simulink model "R7014E_QuadTankSim"  (R2025b)
settings: Solver=ode4  StartTime=0.0  StopTime=2000  FixedStep=0.01  RelTol=1e-3  EnableMultiTasking=on
values from neighbouring files (symbols this model uses):
  A1 = 28    [matlab_workspace.mat]
  a1 = 0.071    [matlab_workspace.mat]
  A2 = 32    [matlab_workspace.mat]
  a2 = 0.057    [matlab_workspace.mat]
  A3 = 28    [matlab_workspace.mat]
  a3 = 0.071    [matlab_workspace.mat]
  A4 = 32    [matlab_workspace.mat]
  a4 = 0.057    [matlab_workspace.mat]
  g = 981    [matlab_workspace.mat]
  G11_den = [62.4182361958 1]    [matlab_workspace.mat]
  G11_num = [0 2.59815908165]    [matlab_workspace.mat]
  G22_den = [90.6440624664 1]    [matlab_workspace.mat]
  G22_num = [0 2.84679008684]    [matlab_workspace.mat]
  gamma1 = 0.7    [matlab_workspace.mat]
  gamma1_M = 0.7    [matlab_workspace.mat]
  gamma2 = 0.6    [matlab_workspace.mat]
  gamma2_M = 0.6    [matlab_workspace.mat]
  h1_init = 12.3    [matlab_workspace.mat]
  h2_init = 12.8    [matlab_workspace.mat]
  h3_init = 1.6    [matlab_workspace.mat]
  h4_init = 1.4    [matlab_workspace.mat]
  k1 = 3.33    [matlab_workspace.mat]
  k1_M = 3.33    [matlab_workspace.mat]
  k2 = 3.35    [matlab_workspace.mat]
  k2_M = 3.35    [matlab_workspace.mat]
  Q = gram(G_Pm,'o')    [Gramians_test.m]    (also in matlab_workspace.mat = [1e-08  0  0; 0  1e-08  0; 0  0  10])
  Q11_den = [23.3834317349 15.5889544899 2.59815908165]    [matlab_workspace.mat]
  Q11_num = [0 62.4182361958 1]    [matlab_workspace.mat]
  Q22_den = [25.6211107815 17.080740521 2.84679008684]    [matlab_workspace.mat]
  Q22_num = [0 90.6440624664 1]    [matlab_workspace.mat]
  R = 0.1    [matlab_workspace.mat]
  Ts = 0.02    [matlab_workspace.mat]
undefined symbols (not defined in the file or in its folder): sigbuilder_block
Description:
  | Double tank process simulation model
  | V1.0
  | 
  | Author: Wolfgang Birk, LTU
settings Model: MinMaxOverflowLogging=ForceOff  Creator=wolfgang  LastModifiedBy=kaspe
settings SolverCC: AlgebraicLoopSolver=TrustRegion
settings DataIOCC: LimitDataPoints=on  SaveFormat=Array  SignalLoggingSaveFormat=ModelDataLogs  ReturnWorkspaceOutputs=off
settings OptimizationCC: ExpressionDepthLimit=2147483647.0  LifeSpan=inf
settings DebuggingCC: UnderspecifiedInitializationDetection=Classic  MergeDetectMultiDrivingBlocksExec=none  SolverPrmCheckMsg=warning  FcnCallInpInsideContextMsg=warning  UnconnectedInputMsg=warning  UnconnectedOutputMsg=warning  UnconnectedLineMsg=warning  StateNameClashWarn=warning  SFUnexpectedBacktrackingDiag=warning  SFNoUnconditionalDefaultTransitionDiag=warning  SFExecutionAtInitializationDiag=none  ArithmeticOperatorsInVariantConditions=warning
settings HardwareCC: ProdBitPerPointer=32.0  ProdBitPerSizeT=32.0  ProdBitPerPtrDiffT=32.0  ProdLargestAtomicFloat=None  ProdIntDivRoundTo=Undefined  ProdEndianess=Unspecified  ProdWordSize=32.0  ProdHWDeviceType=32-bit Generic
settings ModelReferenceCC: EnableRefExpFcnMdlSchedulingChecks=on  PropagateSignalLabelsOutOfModel=off
settings SFSimCC: SimUseLocalCustomCode=off  CustomCodeUndefinedFunction=UseInterfaceOnly
settings RTWCC: RTWUseLocalCustomCode=off  GPUComputeCapability=3.5
settings CodeAppCC: StateflowObjectComments=on
settings GRTTargetCC: TargetLangStandard=C89/C90 (ANSI)
settings ConfigComp: CovMetricSettings=dw  CovSaveCumulativeToWorkspaceVar=on  CovSaveSingleToWorkspaceVar=on  CovExternalEMLEnable=off

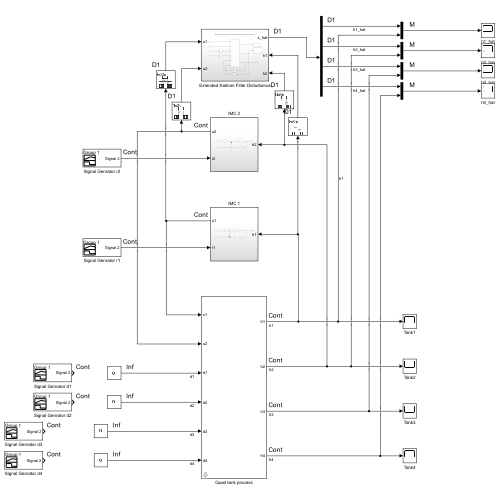
[thumbnail: Simulink's stored preview of the top-level diagram]
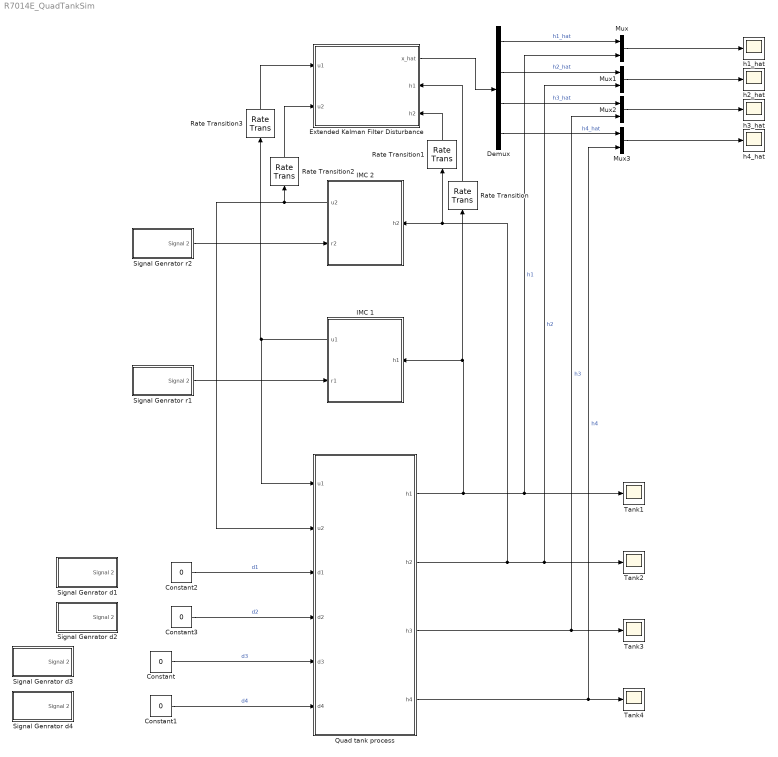
== system R7014E_QuadTankSim ==
  Constant{,1..3} (4 alike) : Constant  Value=0
  Demux : Demux
  Extended Kalman Filter Disturbance : Subsystem
      settings: PortSchema="{\"entries\":[{\"content\":{\"sides\":[{\"content\":{\"connectorIds\":[\"In1\",\"In2\"]},\"type\":\"ConnectorPlacement.EquallySpacedRectSide\",\"uuid\":\"65fe89cb-b391-4b62-a3a2-a3476ef8bc40\"},{\"content\":{\"connectorIds\":[\"Out1\",\"In3\",\"In4\"],\"side\":\"RIGHT\"},\"type\":\"ConnectorPlacement.EquallySpacedRectSide\",\"uuid\":\"bbc6305a-5625-4988-a68f-cd512a800022\"},{\"content\":{\"side\":\"TOP\"},\"type\":\"ConnectorPlacement.EquallySpacedRectSide\",\"uuid\":\"302c5684-92d4-4b6e-95b2-967c1f4e7e8f\"},{\"content\":{\"side\":\"BOTTOM\"},\"type\":\"ConnectorPlacement.EquallySpacedRectSide\",\"uuid\":\"8db0117f-7782-4a07-8d3a-766a48ad4692\"}]},\"type\":\"ConnectorPlacement.EquallySpacedConnector\",\"uuid\":\"a95b63f5-df7a-433e-a941-cc1845937f8d\"}],\"packageUris\":[\"http://schema.mathworks.com/mf0/Connector/R2020b\"],\"version\":\"1.0\"}"
  IMC 1 : Subsystem
      settings: PortSchema="{\"entries\":[{\"content\":{\"sides\":[{\"content\":{\"connectorIds\":[\"In1\"]},\"type\":\"ConnectorPlacement.EquallySpacedRectSide\",\"uuid\":\"4852cb48-3dbe-49d3-b52d-1f2b66e5782f\"},{\"content\":{\"connectorIds\":[\"Out1\",\"In2\"],\"side\":\"RIGHT\"},\"type\":\"ConnectorPlacement.EquallySpacedRectSide\",\"uuid\":\"9cc98c43-55ba-47ec-98d3-91ba0e651a74\"},{\"content\":{\"side\":\"TOP\"},\"type\":\"ConnectorPlacement.EquallySpacedRectSide\",\"uuid\":\"0e4ead2b-996b-4075-849e-a6886983cab4\"},{\"content\":{\"side\":\"BOTTOM\"},\"type\":\"ConnectorPlacement.EquallySpacedRectSide\",\"uuid\":\"443cd1da-2b11-4b7b-ba12-e267a6b444a4\"}]},\"type\":\"ConnectorPlacement.EquallySpacedConnector\",\"uuid\":\"d0829c27-0885-4d8f-a753-a80de6d2ea12\"}],\"packageUris\":[\"http://schema.mathworks.com/mf0/Connector/R2020b\"],\"version\":\"1.0\"}"
  IMC 2 : Subsystem
      settings: PortSchema="{\"entries\":[{\"content\":{\"sides\":[{\"content\":{\"connectorIds\":[\"In1\"]},\"type\":\"ConnectorPlacement.EquallySpacedRectSide\",\"uuid\":\"4852cb48-3dbe-49d3-b52d-1f2b66e5782f\"},{\"content\":{\"connectorIds\":[\"Out1\",\"In2\"],\"side\":\"RIGHT\"},\"type\":\"ConnectorPlacement.EquallySpacedRectSide\",\"uuid\":\"9cc98c43-55ba-47ec-98d3-91ba0e651a74\"},{\"content\":{\"side\":\"TOP\"},\"type\":\"ConnectorPlacement.EquallySpacedRectSide\",\"uuid\":\"0e4ead2b-996b-4075-849e-a6886983cab4\"},{\"content\":{\"side\":\"BOTTOM\"},\"type\":\"ConnectorPlacement.EquallySpacedRectSide\",\"uuid\":\"84a55638-02cd-431e-8938-8d2f80adb47b\"}]},\"type\":\"ConnectorPlacement.EquallySpacedConnector\",\"uuid\":\"d0829c27-0885-4d8f-a753-a80de6d2ea12\"}],\"packageUris\":[\"http://schema.mathworks.com/mf0/Connector/R2020b\"],\"version\":\"1.0\"}"
  Mux{,1..3} (4 alike) : Mux  Inputs=2
  Quad tank process : Subsystem  mask{hmax=20, A1=A1, ao1=a1, h10=0, A2=A2, ao2=a2, h20=0, A3=A3, ao3=a3, h30=0, A4=A4, ao4=a4, h40=0, k1=k1_M, k2=k2_M, gamma1=gamma1_M, gamma2=gamma2_M}
      mask prompts: hmax "Tank height (cm)"; A1 "Tank area (cm^2)"; ao1 "Opening area (cm^2)"; h10 "Initial level (cm)"; A2 "Tank area (cm^2)"; ao2 "Opening area (cm^2)"; h20 "Initial level (cm)"; A3 "Tank area (cm^2)"; ao3 "Opening area (cm^2)"; h30 "Initial level (cm)"; A4 "Tank area (cm^2)"; ao4 "Opening area (cm^2)"; h40 "Initial level (cm)"; k1 "Pump1 gain (cm^3/V/s)"; k2 "Pump2 gain (cm^3/V/s)"; gamma1 "Split valve gamma 1"; gamma2 "Split valve gamma 2"
      mask help: Double tank process parameters
      mask DialogControl Container3 Prompt: General parameters
      mask DialogControl ParameterGroupVar Prompt: Tank 1
      mask DialogControl ParameterGroupVar_copy_copy_copy Prompt: Tank 2
      mask DialogControl ParameterGroupVar_copy_copy Prompt: Tank 3
      mask DialogControl ParameterGroupVar_copy Prompt: Tank 4
      mask DialogControl Container4 Prompt: Pump parameters
  Rate Transition : RateTransition  InitialCondition=h1_init  OutPortSampleTime=Ts
  Rate Transition1 : RateTransition  InitialCondition=h2_init  OutPortSampleTime=Ts
  Rate Transition2 : RateTransition  InitialCondition=h2_init  OutPortSampleTime=Ts
  Rate Transition3 : RateTransition  InitialCondition=h2_init  OutPortSampleTime=Ts
  Signal Genrator d1 : Subsystem  Tag=STV Subsys  LoadFcn=sigbuilder_block('load');  StartFcn=sigbuilder_block('start');  StopFcn=sigbuilder_block('stop');  ClipboardFcn=sigbuilder_block('clipboard');  mask(Sigbuilder block){tuvar=[0:10]}
      mask help: Simulink:masks:SigbuilderBlock_MD
      mask init:
      | if ~strcmp(get_param(bdroot(gcbh),'SimulationStatus'),'stopped') tuvar = sigbuilder_block('maskInit'); end
      settings: CopyFcn=sigbuilder_block('copy');  DeleteFcn=sigbuilder_block('delete');  ModelCloseFcn=sigbuilder_block('modelClose');  PreSaveFcn=sigbuilder_block('preSave');  PauseFcn=sigbuilder_block('pause');  ContinueFcn=sigbuilder_block('continue');  NameChangeFcn=sigbuilder_block('namechange');  OpenFcn=sigbuilder_block('open',[335.25 1257.75 630.75 369 ]);  CloseFcn=sigbuilder_block('close');
      mask Display: plot(0, 0, 100, 100,[2, 2, 32, 32, 2], [68, 8, 8, 68, 68],[32, 2], [38, 38], [32, 19, 2],[53, 60, 44], [32, 17, 17, 2],[16, 16, 31, 31]);txt = getActiveGroup(gcbh);text(2, 100, txt,'verticalAlignment', 'top');
  Signal Genrator d2 : Subsystem  Tag=STV Subsys  LoadFcn=sigbuilder_block('load');  StartFcn=sigbuilder_block('start');  StopFcn=sigbuilder_block('stop');  ClipboardFcn=sigbuilder_block('clipboard');  mask(Sigbuilder block){tuvar=[0:10]}
      mask help: Simulink:masks:SigbuilderBlock_MD
      mask init:
      | if ~strcmp(get_param(bdroot(gcbh),'SimulationStatus'),'stopped') tuvar = sigbuilder_block('maskInit'); end
      settings: CopyFcn=sigbuilder_block('copy');  DeleteFcn=sigbuilder_block('delete');  ModelCloseFcn=sigbuilder_block('modelClose');  PreSaveFcn=sigbuilder_block('preSave');  PauseFcn=sigbuilder_block('pause');  ContinueFcn=sigbuilder_block('continue');  NameChangeFcn=sigbuilder_block('namechange');  OpenFcn=sigbuilder_block('open',[609.75 1396.5 630.75 369 ]);  CloseFcn=sigbuilder_block('close');
      mask Display: plot(0, 0, 100, 100,[2, 2, 32, 32, 2], [68, 8, 8, 68, 68],[32, 2], [38, 38], [32, 19, 2],[53, 60, 44], [32, 17, 17, 2],[16, 16, 31, 31]);txt = getActiveGroup(gcbh);text(2, 100, txt,'verticalAlignment', 'top');
  Signal Genrator d3 : Subsystem  Tag=STV Subsys  LoadFcn=sigbuilder_block('load');  StartFcn=sigbuilder_block('start');  StopFcn=sigbuilder_block('stop');  ClipboardFcn=sigbuilder_block('clipboard');  mask(Sigbuilder block){tuvar=[0:10]}
      mask help: Simulink:masks:SigbuilderBlock_MD
      mask init:
      | if ~strcmp(get_param(bdroot(gcbh),'SimulationStatus'),'stopped') tuvar = sigbuilder_block('maskInit'); end
      settings: CopyFcn=sigbuilder_block('copy');  DeleteFcn=sigbuilder_block('delete');  ModelCloseFcn=sigbuilder_block('modelClose');  PreSaveFcn=sigbuilder_block('preSave');  PauseFcn=sigbuilder_block('pause');  ContinueFcn=sigbuilder_block('continue');  NameChangeFcn=sigbuilder_block('namechange');  OpenFcn=sigbuilder_block('open',[603.75 1322.25 630.75 369 ]);  CloseFcn=sigbuilder_block('close');
      mask Display: plot(0, 0, 100, 100,[2, 2, 32, 32, 2], [68, 8, 8, 68, 68],[32, 2], [38, 38], [32, 19, 2],[53, 60, 44], [32, 17, 17, 2],[16, 16, 31, 31]);txt = getActiveGroup(gcbh);text(2, 100, txt,'verticalAlignment', 'top');
  Signal Genrator d4 : Subsystem  Tag=STV Subsys  LoadFcn=sigbuilder_block('load');  StartFcn=sigbuilder_block('start');  StopFcn=sigbuilder_block('stop');  ClipboardFcn=sigbuilder_block('clipboard');  mask(Sigbuilder block){tuvar=[0:10]}
      mask help: Simulink:masks:SigbuilderBlock_MD
      mask init:
      | if ~strcmp(get_param(bdroot(gcbh),'SimulationStatus'),'stopped') tuvar = sigbuilder_block('maskInit'); end
      settings: CopyFcn=sigbuilder_block('copy');  DeleteFcn=sigbuilder_block('delete');  ModelCloseFcn=sigbuilder_block('modelClose');  PreSaveFcn=sigbuilder_block('preSave');  PauseFcn=sigbuilder_block('pause');  ContinueFcn=sigbuilder_block('continue');  NameChangeFcn=sigbuilder_block('namechange');  OpenFcn=sigbuilder_block('open',[271.5 378 630.75 369 ]);  CloseFcn=sigbuilder_block('close');
      mask Display: plot(0, 0, 100, 100,[2, 2, 32, 32, 2], [68, 8, 8, 68, 68],[32, 2], [38, 38], [32, 19, 2],[53, 60, 44], [32, 17, 17, 2],[16, 16, 31, 31]);txt = getActiveGroup(gcbh);text(2, 100, txt,'verticalAlignment', 'top');
  Signal Genrator r1 : Subsystem  Tag=STV Subsys  LoadFcn=sigbuilder_block('load');  StartFcn=sigbuilder_block('start');  StopFcn=sigbuilder_block('stop');  ClipboardFcn=sigbuilder_block('clipboard');  mask(Sigbuilder block){tuvar=[0:10]}
      mask help: Simulink:masks:SigbuilderBlock_MD
      mask init:
      | if ~strcmp(get_param(bdroot(gcbh),'SimulationStatus'),'stopped') tuvar = sigbuilder_block('maskInit'); end
      settings: CopyFcn=sigbuilder_block('copy');  DeleteFcn=sigbuilder_block('delete');  ModelCloseFcn=sigbuilder_block('modelClose');  PreSaveFcn=sigbuilder_block('preSave');  PauseFcn=sigbuilder_block('pause');  ContinueFcn=sigbuilder_block('continue');  NameChangeFcn=sigbuilder_block('namechange');  OpenFcn=sigbuilder_block('open',[271.5 378 630.75 369 ]);  CloseFcn=sigbuilder_block('close');
      mask Display: plot(0, 0, 100, 100,[2, 2, 32, 32, 2], [68, 8, 8, 68, 68],[32, 2], [38, 38], [32, 19, 2],[53, 60, 44], [32, 17, 17, 2],[16, 16, 31, 31]);txt = getActiveGroup(gcbh);text(2, 100, txt,'verticalAlignment', 'top');
  Signal Genrator r2 : Subsystem  Tag=STV Subsys  LoadFcn=sigbuilder_block('load');  StartFcn=sigbuilder_block('start');  StopFcn=sigbuilder_block('stop');  ClipboardFcn=sigbuilder_block('clipboard');  mask(Sigbuilder block){tuvar=[0:10]}
      mask help: Simulink:masks:SigbuilderBlock_MD
      mask init:
      | if ~strcmp(get_param(bdroot(gcbh),'SimulationStatus'),'stopped') tuvar = sigbuilder_block('maskInit'); end
      settings: CopyFcn=sigbuilder_block('copy');  DeleteFcn=sigbuilder_block('delete');  ModelCloseFcn=sigbuilder_block('modelClose');  PreSaveFcn=sigbuilder_block('preSave');  PauseFcn=sigbuilder_block('pause');  ContinueFcn=sigbuilder_block('continue');  NameChangeFcn=sigbuilder_block('namechange');  OpenFcn=sigbuilder_block('open',[271.5 378 630.75 369 ]);  CloseFcn=sigbuilder_block('close');
      mask Display: plot(0, 0, 100, 100,[2, 2, 32, 32, 2], [68, 8, 8, 68, 68],[32, 2], [38, 38], [32, 19, 2],[53, 60, 44], [32, 17, 17, 2],[16, 16, 31, 31]);txt = getActiveGroup(gcbh);text(2, 100, txt,'verticalAlignment', 'top');
  Tank{1..4} (4 alike) : Scope
      Tank1 settings: TimeSpan=100  ActiveDisplayYMinimum=-1.8059795256397659  ActiveDisplayYMaximum=16.253815730757896
      Tank2 settings: TimeSpan=100  ActiveDisplayYMinimum=-1.9584679823736892  ActiveDisplayYMaximum=17.626211841363208  DataLoggingVariableName=ScopeData3
      Tank3 settings: TimeSpan=100  ActiveDisplayYMinimum=1.57505  ActiveDisplayYMaximum=1.66866
      Tank4 settings: TimeSpan=100  ActiveDisplayYMinimum=1.35987  ActiveDisplayYMaximum=1.45363  DataLoggingVariableName=ScopeData2
  h1_hat : Scope
      settings: ActiveDisplayYMinimum=-1.8062354240144811  ActiveDisplayYMaximum=16.256118816130336  DataLoggingVariableName=ScopeData4
  h2_hat : Scope
      settings: ActiveDisplayYMinimum=-1.8062354240144811  ActiveDisplayYMaximum=16.256118816130336  DataLoggingVariableName=ScopeData5
  h3_hat : Scope
      settings: ActiveDisplayYMinimum=-1.8062354240144811  ActiveDisplayYMaximum=16.256118816130336  DataLoggingVariableName=ScopeData6
  h4_hat : Scope
      settings: ActiveDisplayYMinimum=-1.8062354240144811  ActiveDisplayYMaximum=16.256118816130336  DataLoggingVariableName=ScopeData7
  wires:
  Quad tank process/3(h3) -> Mux2/2, Tank3/1  "h3"
  Quad tank process/1(h1) -> IMC 1/1(h1), Rate Transition/1, Mux/2, Tank1/1  "h1"
  Constant2/1 -> Quad tank process/3(d1)  "d1"
  Constant3/1 -> Quad tank process/4(d2)  "d2"
  Constant/1 -> Quad tank process/5(d3)  "d3"
  Constant1/1 -> Quad tank process/6(d4)  "d4"
  Quad tank process/2(h2) -> Mux1/2, Tank2/1, IMC 2/1(h2), Rate Transition1/1  "h2"
  Quad tank process/4(h4) -> Mux3/2, Tank4/1  "h4"
  IMC 1/1(u1) -> Rate Transition3/1, Quad tank process/1(u1)
  Signal Genrator r1/1(Signal 2) -> IMC 1/2(r1)
  Signal Genrator r2/1(Signal 2) -> IMC 2/2(r2)
  IMC 2/1(u2) -> Quad tank process/2(u2), Rate Transition2/1
  Rate Transition/1 -> Extended Kalman Filter Disturbance/3(h1)
  Rate Transition1/1 -> Extended Kalman Filter Disturbance/4(h2)
  Rate Transition2/1 -> Extended Kalman Filter Disturbance/2(u2)
  Rate Transition3/1 -> Extended Kalman Filter Disturbance/1(u1)
  Extended Kalman Filter Disturbance/1(x_hat) -> Demux/1
  Demux/1 -> Mux/1  "h1_hat"
  Mux/1 -> h1_hat/1
  Demux/2 -> Mux1/1  "h2_hat"
  Demux/3 -> Mux2/1  "h3_hat"
  Demux/4 -> Mux3/1  "h4_hat"
  Mux1/1 -> h2_hat/1
  Mux2/1 -> h3_hat/1
  Mux3/1 -> h4_hat/1

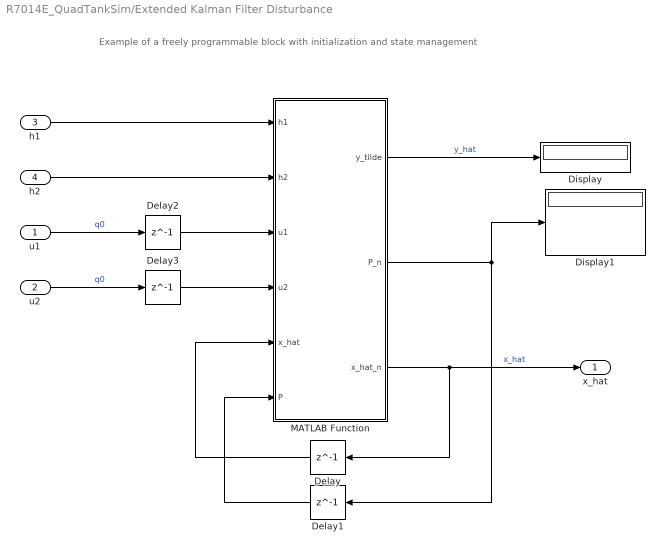
== system R7014E_QuadTankSim/Extended Kalman Filter Disturbance ==
  note: Example of a freely programmable block with initialization and state management
  u1 : Inport
  u2 : Inport  Port=2
  h1 : Inport  Port=3
  h2 : Inport  Port=4
  Delay : Delay  DelayLength=1  InitialCondition=[h1_init, h2_init, h3_init, h4_init]
  Delay1 : Delay  DelayLength=1  InitialCondition=zeros(4)
  Delay2 : Delay  DelayLength=1  InitialCondition=0
  Delay3 : Delay  DelayLength=1  InitialCondition=0
  Display : Display
  Display1 : Display
  MATLAB Function : MATLAB Function  TreatAsAtomicUnit=on
  x_hat : Outport
  wires:
  Delay/1 -> MATLAB Function/5(x_hat)
  MATLAB Function/1(y_tilde) -> Display/1  "y_hat"
  MATLAB Function/2(P_n) -> Display1/1, Delay1/1
  Delay1/1 -> MATLAB Function/6(P)
  u1/1 -> Delay2/1  "q0"
  MATLAB Function/3(x_hat_n) -> x_hat/1, Delay/1  "x_hat"
  Delay2/1 -> MATLAB Function/3(u1)
  Delay3/1 -> MATLAB Function/4(u2)
  u2/1 -> Delay3/1  "q0"
  h2/1 -> MATLAB Function/2(h2)
  h1/1 -> MATLAB Function/1(h1)

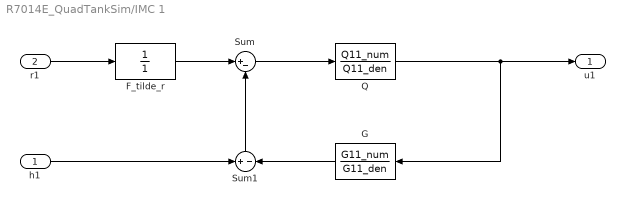
== system R7014E_QuadTankSim/IMC 1 ==
  h1 : Inport
  r1 : Inport  Port=2
  F_tilde_r : TransferFcn  Denominator=[1]
  G : TransferFcn  Numerator=G11_num  Denominator=G11_den
  Q : TransferFcn  Numerator=Q11_num  Denominator=Q11_den
  Sum : Sum  Inputs=|+-
  Sum1 : Sum  Inputs=+|-
  u1 : Outport
  wires:
  F_tilde_r/1 -> Sum/1
  r1/1 -> F_tilde_r/1
  Sum/1 -> Q/1
  Sum1/1 -> Sum/2
  Q/1 -> G/1, u1/1
  G/1 -> Sum1/2
  h1/1 -> Sum1/1

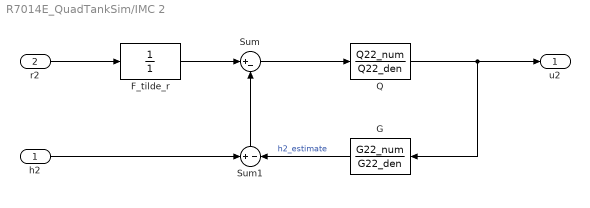
== system R7014E_QuadTankSim/IMC 2 ==
  h2 : Inport
  r2 : Inport  Port=2
  F_tilde_r : TransferFcn  Denominator=[1]
  G : TransferFcn  Numerator=G22_num  Denominator=G22_den
  Q : TransferFcn  Numerator=Q22_num  Denominator=Q22_den
  Sum : Sum  Inputs=|+-
  Sum1 : Sum  Inputs=+|-
  u2 : Outport
  wires:
  F_tilde_r/1 -> Sum/1
  r2/1 -> F_tilde_r/1
  Sum/1 -> Q/1
  Sum1/1 -> Sum/2
  Q/1 -> u2/1, G/1
  h2/1 -> Sum1/1
  G/1 -> Sum1/2  "h2_estimate"

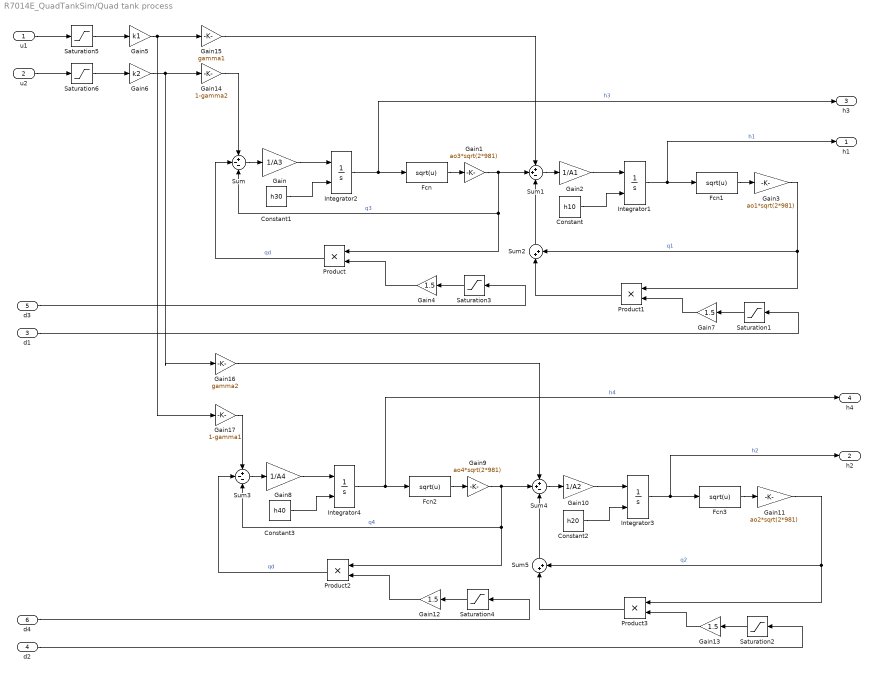
== system R7014E_QuadTankSim/Quad tank process ==
  u1 : Inport
  u2 : Inport  Port=2
  d1 : Inport  Port=3
  d2 : Inport  Port=4
  d3 : Inport  Port=5
  d4 : Inport  Port=6
  Constant : Constant  Value=h10
  Constant1 : Constant  Value=h30
  Constant2 : Constant  Value=h20
  Constant3 : Constant  Value=h40
  Fcn{,1..3} (4 alike) : Fcn  Expr=sqrt(u)
  Gain : Gain  Gain=1/A3
  Gain1 : Gain  Gain=ao3*sqrt(2*981)
  Gain10 : Gain  Gain=1/A2
  Gain11 : Gain  Gain=ao2*sqrt(2*981)
  Gain{4,7,12..13} (4 alike) : Gain  Gain=1.5
  Gain14 : Gain  Gain=1-gamma2
  Gain15 : Gain  Gain=gamma1
  Gain16 : Gain  Gain=gamma2
  Gain17 : Gain  Gain=1-gamma1
  Gain2 : Gain  Gain=1/A1
  Gain3 : Gain  Gain=ao1*sqrt(2*981)
  Gain5 : Gain  Gain=k1
  Gain6 : Gain  Gain=k2
  Gain8 : Gain  Gain=1/A4
  Gain9 : Gain  Gain=ao4*sqrt(2*981)
  Integrator{1..4} (4 alike) : Integrator  InitialConditionSource=external  LimitOutput=on  UpperSaturationLimit=hmax  LowerSaturationLimit=0
  Product{,1..3} (4 alike) : Product  RndMeth=Zero
  Saturation{1..4} (4 alike) : Saturate  UpperLimit=1  LowerLimit=0
  Saturation5 : Saturate  UpperLimit=10  LowerLimit=0
  Saturation6 : Saturate  UpperLimit=10  LowerLimit=0
  Sum : Sum  Inputs=+--
  Sum1 : Sum  Inputs=++-
  Sum2 : Sum  Inputs=|++
  Sum3 : Sum  Inputs=+--
  Sum4 : Sum  Inputs=++-
  Sum5 : Sum  Inputs=|++
  h1 : Outport  VectorParamsAs1DForOutWhenUnconnected=off
  h2 : Outport  Port=2  VectorParamsAs1DForOutWhenUnconnected=off
  h3 : Outport  Port=3  VectorParamsAs1DForOutWhenUnconnected=off
  h4 : Outport  Port=4  VectorParamsAs1DForOutWhenUnconnected=off
  wires:
  Sum/1 -> Gain/1
  Gain/1 -> Integrator2/1
  Fcn/1 -> Gain1/1
  Gain1/1 -> Product/1, Sum/3, Sum1/2  "q3"
  Sum1/1 -> Gain2/1
  Gain2/1 -> Integrator1/1
  Fcn1/1 -> Gain3/1
  Integrator2/1 -> h3/1, Fcn/1  "h3"
  Product/1 -> Sum/2  "qd"
  d3/1 -> Saturation3/1
  Integrator1/1 -> h1/1, Fcn1/1  "h1"
  Saturation3/1 -> Gain4/1
  Gain4/1 -> Product/2
  u1/1 -> Saturation5/1
  Constant/1 -> Integrator1/2
  Constant1/1 -> Integrator2/2
  u2/1 -> Saturation6/1
  Gain5/1 -> Gain17/1, Gain15/1
  Sum2/1 -> Sum1/3
  Gain3/1 -> Product1/1, Sum2/2  "q1"
  Gain7/1 -> Product1/2
  Saturation1/1 -> Gain7/1
  d1/1 -> Saturation1/1
  Product1/1 -> Sum2/1
  Product3/1 -> Sum5/1
  d2/1 -> Saturation2/1
  Saturation2/1 -> Gain13/1
  Gain13/1 -> Product3/2
  Gain11/1 -> Sum5/2, Product3/1  "q2"
  Sum5/1 -> Sum4/3
  Constant3/1 -> Integrator4/2
  Constant2/1 -> Integrator3/2
  Gain12/1 -> Product2/2
  Saturation4/1 -> Gain12/1
  Integrator3/1 -> Fcn3/1, h2/1  "h2"
  d4/1 -> Saturation4/1
  Product2/1 -> Sum3/2  "qd"
  Integrator4/1 -> h4/1, Fcn2/1  "h4"
  Fcn3/1 -> Gain11/1
  Gain10/1 -> Integrator3/1
  Sum4/1 -> Gain10/1
  Gain9/1 -> Sum4/2, Sum3/3, Product2/1  "q4"
  Fcn2/1 -> Gain9/1
  Gain8/1 -> Integrator4/1
  Sum3/1 -> Gain8/1
  Gain14/1 -> Sum/1
  Gain15/1 -> Sum1/1
  Gain6/1 -> Gain16/1, Gain14/1
  Gain16/1 -> Sum4/1
  Gain17/1 -> Sum3/1
  Saturation5/1 -> Gain5/1
  Saturation6/1 -> Gain6/1

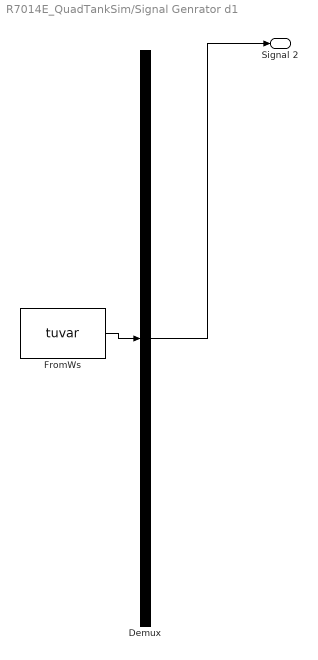
== system R7014E_QuadTankSim/Signal Genrator d1 ==
  Demux : Demux  Tag=STV Demux  Outputs=1
      settings: DisplayOption=none
  FromWs : FromWorkspace  Tag=STV FromWs  VariableName=tuvar
      SigBuilderData=|
      | common.afterFinalStr = 'Extrapolate'
      | common.sampleTime = 0
      | dataSet.timeRange = [0 2000]
      | dataSet.name = 'Group 1'
      | sbobj.Groups.Name = 'Group 1'
      | sbobj.Groups.Signals.Name = 'Signal 2'
      | sbobj.Groups.Signals.XData = [0 1400 1400 2000]
      | sbobj.Groups.Signals.YData = [0.5 0.5 0.75 0.75]
      | sbobj.Groups.TimeRange = [0 2000]
  Signal 2 : Outport  Tag=STV Outport
  wires:
  FromWs/1 -> Demux/1
  Demux/1 -> Signal 2/1

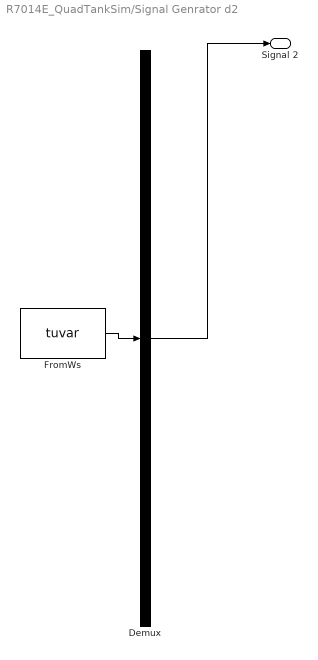
== system R7014E_QuadTankSim/Signal Genrator d2 ==
  Demux : Demux  Tag=STV Demux  Outputs=1
      settings: DisplayOption=none
  FromWs : FromWorkspace  Tag=STV FromWs  VariableName=tuvar
      SigBuilderData=|
      | common.afterFinalStr = 'Extrapolate'
      | common.sampleTime = 0
      | dataSet.timeRange = [0 2000]
      | dataSet.name = 'Group 1'
      | sbobj.Groups.Name = 'Group 1'
      | sbobj.Groups.Signals.Name = 'Signal 2'
      | sbobj.Groups.Signals.XData = [0 1400 1400 2000]
      | sbobj.Groups.Signals.YData = [0.5 0.5 0.25 0.25]
      | sbobj.Groups.TimeRange = [0 2000]
  Signal 2 : Outport  Tag=STV Outport
  wires:
  FromWs/1 -> Demux/1
  Demux/1 -> Signal 2/1

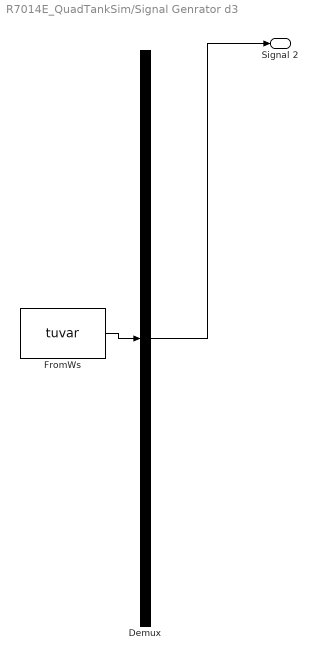
== system R7014E_QuadTankSim/Signal Genrator d3 ==
  Demux : Demux  Tag=STV Demux  Outputs=1
      settings: DisplayOption=none
  FromWs : FromWorkspace  Tag=STV FromWs  VariableName=tuvar
      SigBuilderData=|
      | common.afterFinalStr = 'Extrapolate'
      | common.sampleTime = 0
      | dataSet.timeRange = [0 2000]
      | dataSet.name = 'Group 1'
      | sbobj.Groups.Name = 'Group 1'
      | sbobj.Groups.Signals.Name = 'Signal 2'
      | sbobj.Groups.Signals.XData = [0 800 800 2000]
      | sbobj.Groups.Signals.YData = [12.3 12.3 14.3 14.3]
      | sbobj.Groups.TimeRange = [0 2000]
  Signal 2 : Outport  Tag=STV Outport
  wires:
  FromWs/1 -> Demux/1
  Demux/1 -> Signal 2/1

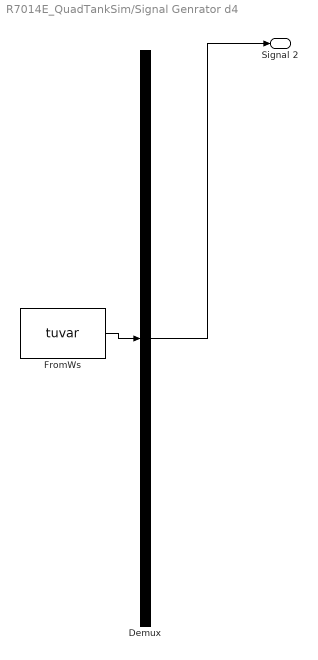
== system R7014E_QuadTankSim/Signal Genrator d4 ==
  Demux : Demux  Tag=STV Demux  Outputs=1
      settings: DisplayOption=none
  FromWs : FromWorkspace  Tag=STV FromWs  VariableName=tuvar
      SigBuilderData=|
      | common.afterFinalStr = 'Extrapolate'
      | common.sampleTime = 0
      | dataSet.timeRange = [0 2000]
      | dataSet.name = 'Group 1'
      | sbobj.Groups.Name = 'Group 1'
      | sbobj.Groups.Signals.Name = 'Signal 2'
      | sbobj.Groups.Signals.XData = [0 800 800 2000]
      | sbobj.Groups.Signals.YData = [12.3 12.3 14.3 14.3]
      | sbobj.Groups.TimeRange = [0 2000]
  Signal 2 : Outport  Tag=STV Outport
  wires:
  FromWs/1 -> Demux/1
  Demux/1 -> Signal 2/1

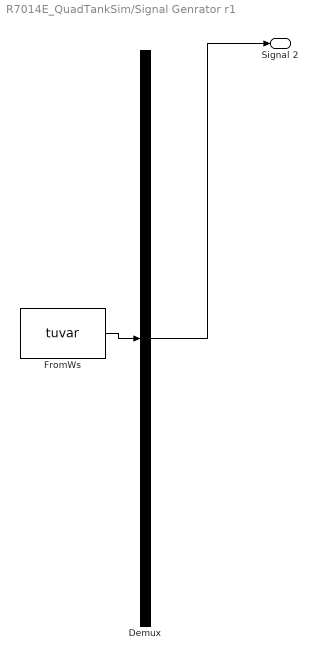
== system R7014E_QuadTankSim/Signal Genrator r1 ==
  Demux : Demux  Tag=STV Demux  Outputs=1
      settings: DisplayOption=none
  FromWs : FromWorkspace  Tag=STV FromWs  VariableName=tuvar
      SigBuilderData=|
      | common.afterFinalStr = 'Extrapolate'
      | common.sampleTime = 0
      | dataSet.timeRange = [0 2000]
      | dataSet.name = 'Group 1'
      | sbobj.Groups.Name = 'Group 1'
      | sbobj.Groups.Signals.Name = 'Signal 2'
      | sbobj.Groups.Signals.XData = [0 800 800 2000]
      | sbobj.Groups.Signals.YData = [12.3 12.3 14.3 14.3]
      | sbobj.Groups.TimeRange = [0 2000]
  Signal 2 : Outport  Tag=STV Outport
  wires:
  FromWs/1 -> Demux/1
  Demux/1 -> Signal 2/1

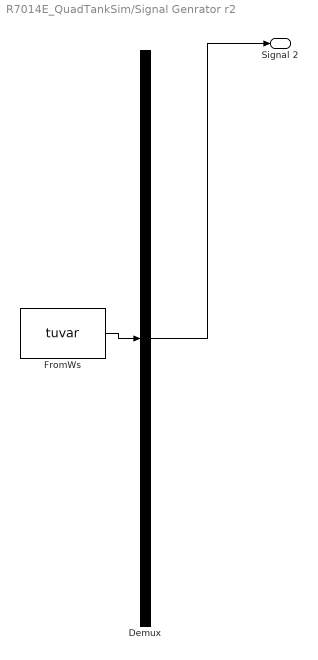
== system R7014E_QuadTankSim/Signal Genrator r2 ==
  Demux : Demux  Tag=STV Demux  Outputs=1
      settings: DisplayOption=none
  FromWs : FromWorkspace  Tag=STV FromWs  VariableName=tuvar
      SigBuilderData=|
      | common.afterFinalStr = 'Extrapolate'
      | common.sampleTime = 0
      | dataSet.timeRange = [0 2000]
      | dataSet.name = 'Group 1'
      | sbobj.Groups.Name = 'Group 1'
      | sbobj.Groups.Signals.Name = 'Signal 2'
      | sbobj.Groups.Signals.XData = [0 800 800 2000]
      | sbobj.Groups.Signals.YData = [12.8 12.8 14.8 14.8]
      | sbobj.Groups.TimeRange = [0 2000]
  Signal 2 : Outport  Tag=STV Outport
  wires:
  FromWs/1 -> Demux/1
  Demux/1 -> Signal 2/1

== matlab function R7014E_QuadTankSim/Extended Kalman Filter Disturbance/MATLAB Function ==
  data: h1 input; h2 input; u1 input; u2 input; x_hat input; y_tilde output; P input; P_n output; x_hat_n output; Q parameter; R parameter; g parameter; Ts parameter; A1 parameter; A2 parameter; A3 parameter; A4 parameter; k1 parameter; k2 parameter; a1 parameter; a2 parameter; a3 parameter; a4 parameter; gamma1 parameter; gamma2 parameter
function [y_tilde, P_n, x_hat_n] = fcn(h1, h2, u1, u2, x_hat, P, Q, R, g, Ts, A1, A2, A3, A4, k1, k2, a1, a2, a3, a4, gamma1, gamma2)

h1_hat = x_hat(1);
h2_hat = x_hat(2);
h3_hat = x_hat(3);
h4_hat = x_hat(4);
Q = eye(4);
% Linearization


% Disturbances (Assumed zero for the filter's internal model unless estimated)
d1 = 0; d2 = 0; d3 = 0; d4 = 0;

% Safety margin to prevent division by zero if a tank empties
epsilon = 1e-6; 

%% Calculate State Jacobian Matrix (A)
A = zeros(4, 4);

A(1,1) = -((a1 + d1) / A1) * sqrt(g / (2 * max(h1_hat, epsilon)));
A(1,3) =  (a3 / A3) * sqrt(g / (2 * max(h3_hat, epsilon)));

A(2,2) = -((a2 + d2) / A2) * sqrt(g / (2 * max(h2_hat, epsilon)));
A(2,4) =  (a4 / A4) * sqrt(g / (2 * max(h4_hat, epsilon)));

A(3,3) = -((a3 + d3) / A3) * sqrt(g / (2 * max(h3_hat, epsilon)));

A(4,4) = -((a4 + d4) / A4) * sqrt(g / (2 * max(h4_hat, epsilon)));

%% Calculate Input Jacobian Matrix (B)
B = zeros(4, 2);

B(1,1) = (gamma1 * k1) / A1;
B(2,2) = (gamma2 * k2) / A2;
B(3,2) = ((1 - gamma2) * k2) / A3;
B(4,1) = ((1 - gamma1) * k1) / A4;

Ad = eye(size(A)) + Ts * A;

% Predict
sqrt1 = sqrt(2*g*max(h1_hat, epsilon));
sqrt2 = sqrt(2*g*max(h2_hat, epsilon));
sqrt3 = sqrt(2*g*max(h3_hat, epsilon));
sqrt4 = sqrt(2*g*max(h4_hat, epsilon));
x_hat_dot = [(-a1-d1)/A1*sqrt1+a3/A3*sqrt3+gamma1/A1*k1*u1;
             (-a2-d2)/A2*sqrt2+a4/A4*sqrt4+gamma2/A2*k2*u2;
             (-a3-d3)/A3*sqrt3+(1-gamma2)/A3*k2*u2;
             (-a4-d4)/A4*sqrt4+(1-gamma1)/A4*k1*u1;];
x_hat_n = x_hat + x_hat_dot .* Ts;
P_n = Ad * P * Ad' + Q;

y = [h1;h2];
C = [1 0 0 0;
     0 1 0 0];

% Update
y_tilde = y - C * x_hat_n;
S = C * P_n * C' + R;
K = P_n * C' * inv(S);
x_hat_n = x_hat_n + K * y_tilde;
P_n = (eye(size(A)) - K * C) * P_n;   
y_tilde = y - C * x_hat_n;
